simulink model "simulink_project3"  (R2025a)
settings: Solver=VariableStepAuto  StartTime=0.0  StopTime=1369  RelTol=1e-3
undefined symbols (not defined in the file or in its folder): vehicle
settings Model: Creator=colto  LastModifiedBy=umar

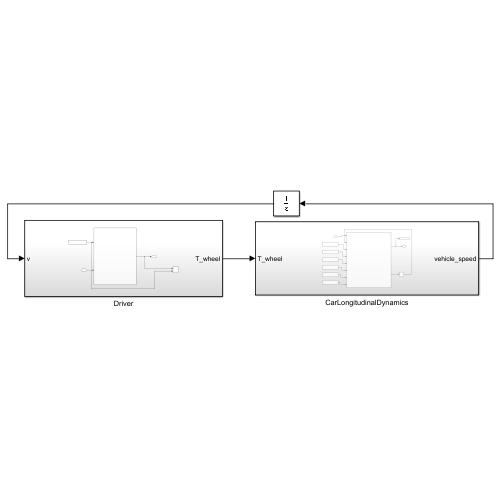
[thumbnail: Simulink's stored preview of the top-level diagram]
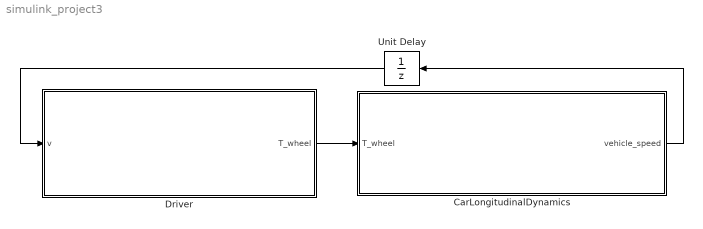
== system simulink_project3 ==
  CarLongitudinalDynamics : Subsystem
  Driver : Subsystem
  Unit Delay : UnitDelay  SampleTime=.1  HasFrameUpgradeWarning=on
  wires:
  Driver/1(T_wheel) -> CarLongitudinalDynamics/1(T_wheel)
  CarLongitudinalDynamics/1(vehicle_speed) -> Unit Delay/1
  Unit Delay/1 -> Driver/1(v)

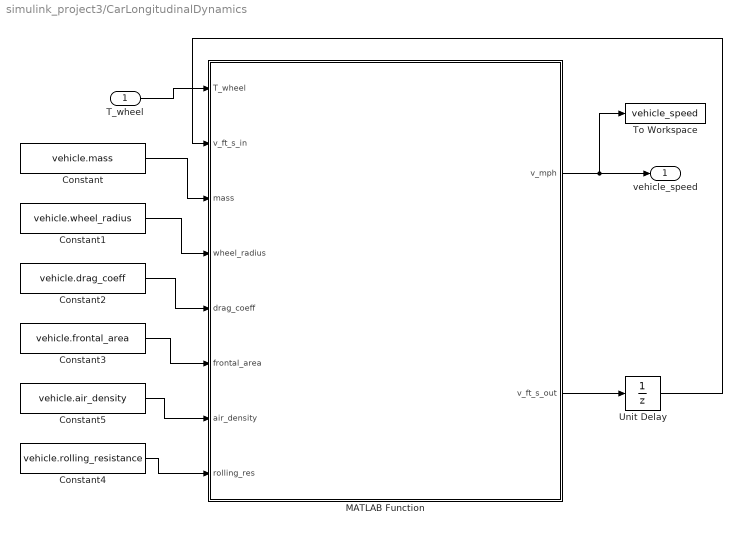
== system simulink_project3/CarLongitudinalDynamics ==
  T_wheel : Inport
  Constant : Constant  Value=vehicle.mass
  Constant1 : Constant  Value=vehicle.wheel_radius
  Constant2 : Constant  Value=vehicle.drag_coeff
  Constant3 : Constant  Value=vehicle.frontal_area
  Constant4 : Constant  Value=vehicle.rolling_resistance
  Constant5 : Constant  Value=vehicle.air_density
  MATLAB Function : MATLAB Function  TreatAsAtomicUnit=on
  To Workspace : ToWorkspace  VariableName=vehicle_speed  SaveFormat=Structure With Time  SampleTime=.1
  Unit Delay : UnitDelay  SampleTime=.1  HasFrameUpgradeWarning=on
  vehicle_speed : Outport
  wires:
  T_wheel/1 -> MATLAB Function/1(T_wheel)
  MATLAB Function/1(v_mph) -> To Workspace/1, vehicle_speed/1
  Constant/1 -> MATLAB Function/3(mass)
  Constant1/1 -> MATLAB Function/4(wheel_radius)
  Constant2/1 -> MATLAB Function/5(drag_coeff)
  Constant3/1 -> MATLAB Function/6(frontal_area)
  Constant5/1 -> MATLAB Function/7(air_density)
  Constant4/1 -> MATLAB Function/8(rolling_res)
  MATLAB Function/2(v_ft_s_out) -> Unit Delay/1
  Unit Delay/1 -> MATLAB Function/2(v_ft_s_in)

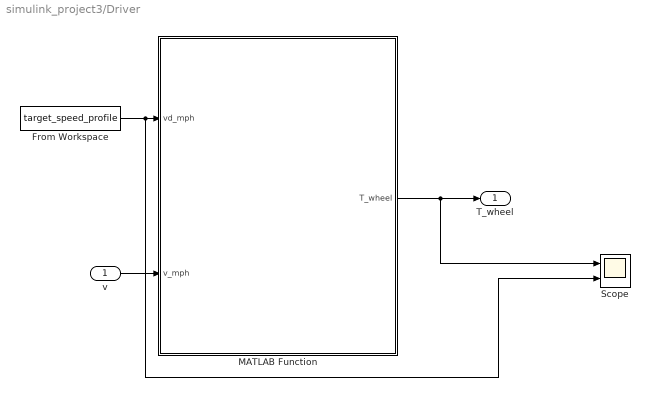
== system simulink_project3/Driver ==
  v : Inport
  From Workspace : FromWorkspace  VariableName=target_speed_profile  SampleTime=.1
  MATLAB Function : MATLAB Function  TreatAsAtomicUnit=on
  Scope : Scope  NumInputPorts=2
      settings: ActiveDisplayYMinimum=-233.93775695006147  ActiveDisplayYMaximum=149.16293330868203
  T_wheel : Outport
  wires:
  MATLAB Function/1(T_wheel) -> Scope/1, T_wheel/1
  v/1 -> MATLAB Function/2(v_mph)
  From Workspace/1 -> Scope/2, MATLAB Function/1(vd_mph)

== matlab function simulink_project3/Driver/MATLAB Function ==
  data: vd_mph input; v_mph input; T_wheel output
function T_wheel = Driver(vd_mph, v_mph)

% Controller gain
Kp = 225;

% Compute error
error = vd_mph - v_mph;

% Compute torque
T_wheel = Kp * error;

% Clamp torque
T_wheel = max(min(T_wheel, 1000), -1000);

== matlab function simulink_project3/CarLongitudinalDynamics/MATLAB Function ==
  data: T_wheel input; v_ft_s_in input; v_mph output; mass input; wheel_radius input; drag_coeff input; frontal_area input; air_density input; rolling_res input; v_ft_s_out output
function [v_mph, v_ft_s_out] = longitudinal_dynamics(T_wheel, v_ft_s_in, mass, wheel_radius, drag_coeff, frontal_area, air_density, rolling_res)

% Constants
g = 32.174;  % ft/s²
dt = 0.1;    % time step

% Resistive forces
F_drag = 0.5 * air_density * drag_coeff * frontal_area * v_ft_s_in^2;
F_roll = rolling_res * mass * g;

% Driving force
F_drive = T_wheel / wheel_radius;

% Net force and acceleration
F_net = F_drive - F_drag - F_roll;
a_ft_s2 = F_net / mass;

% Update velocity
v_ft_s_out = v_ft_s_in + a_ft_s2 * dt;

% Convert to mph
v_mph = v_ft_s_out / 1.46667;
